simulink model "funcTest"  (R2020a)
settings: Solver=VariableStepAuto  StartTime=0.0  StopTime=10.0  RelTol=1e-3
settings Model: Creator=assem  LastModifiedBy=assem

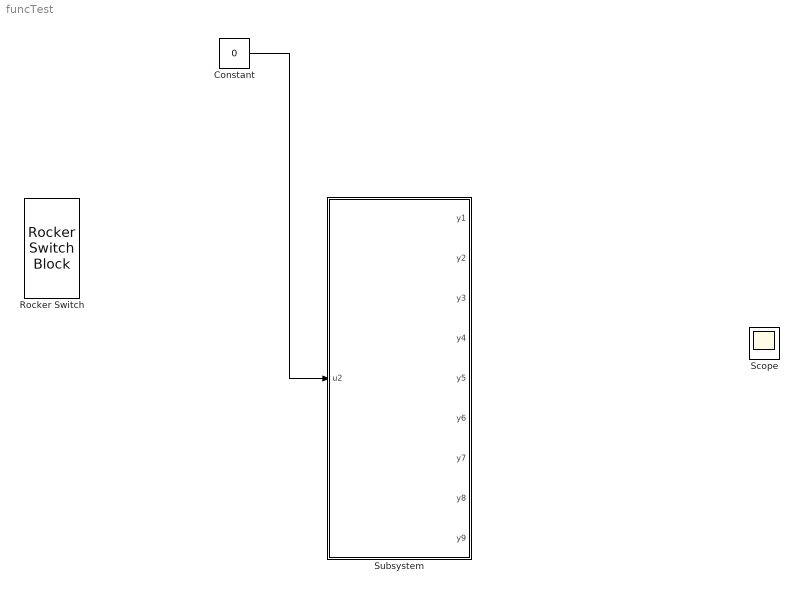
== system funcTest ==
  Constant : Constant  Value=0
  Rocker Switch : RockerSwitchBlock
      settings: Values={{'Off', 'On'}, [0 1]}
  Scope : Scope
  Subsystem : Subsystem
  wires:
  Constant/1 -> Subsystem/1(u2)

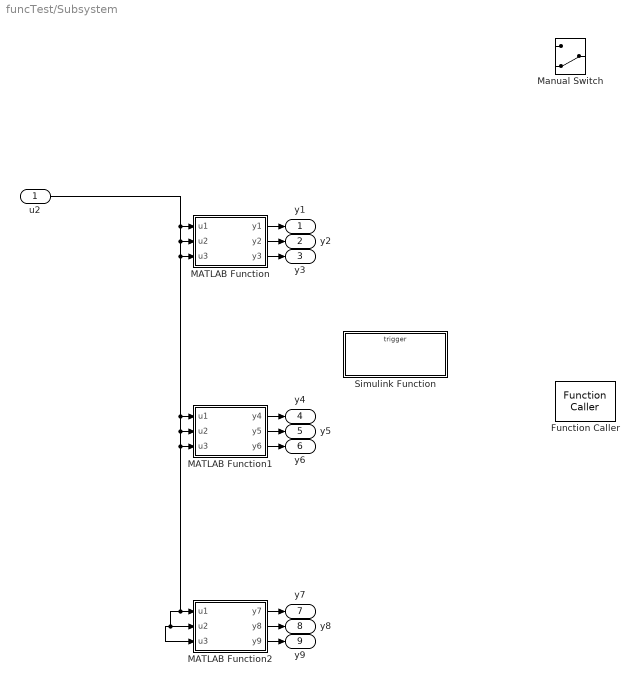
== system funcTest/Subsystem ==
  u2 : Inport
  Function Caller : FunctionCaller  FunctionPrototype=y = f(u)  InputArgumentSpecifications=<Enter example>  OutputArgumentSpecifications=<Enter example>
  MATLAB Function : MATLAB Function  TreatAsAtomicUnit=on
  MATLAB Function1 : MATLAB Function  TreatAsAtomicUnit=on
  MATLAB Function2 : MATLAB Function  TreatAsAtomicUnit=on
  Manual Switch : ManualSwitch  CurrentSetting=0
  Simulink Function : Subsystem  TreatAsAtomicUnit=on
  y1 : Outport
  y2 : Outport  Port=2
  y3 : Outport  Port=3
  y4 : Outport  Port=4
  y5 : Outport  Port=5
  y6 : Outport  Port=6
  y7 : Outport  Port=7
  y8 : Outport  Port=8
  y9 : Outport  Port=9
  wires:
  MATLAB Function2/2(y8) -> y8/1
  MATLAB Function1/1(y4) -> y4/1
  u2/1 -> MATLAB Function2/3(u3), MATLAB Function2/2(u2), MATLAB Function2/1(u1), MATLAB Function1/3(u3), MATLAB Function1/2(u2), MATLAB Function1/1(u1), MATLAB Function/3(u3), MATLAB Function/2(u2), MATLAB Function/1(u1)
  MATLAB Function2/1(y7) -> y7/1
  MATLAB Function2/3(y9) -> y9/1
  MATLAB Function/3(y3) -> y3/1
  MATLAB Function1/2(y5) -> y5/1
  MATLAB Function/1(y1) -> y1/1
  MATLAB Function1/3(y6) -> y6/1
  MATLAB Function/2(y2) -> y2/1

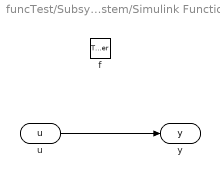
== system funcTest/Subsystem/Simulink Function ==
  f : TriggerPort  TriggerType=function-call  IsSimulinkFunction=on  FunctionName=f  FunctionVisibility=scoped  VariantControl=(inherit)
  u : ArgIn  DisableCoverage=on  ArgumentName=u
  y : ArgOut  DisableCoverage=on  ArgumentName=y
  wires:
  u/1 -> y/1

== matlab function funcTest/Subsystem/MATLAB Function1 ==
  data: u1 input; y4 output; u2 input; u3 input; y5 output; y6 output
function [y4, y5, y6] = fcn2(u1, u2, u3)
    
if (u1 == 1 && u3 == 1)
    y4 = 1;
    y5 = 0;
    y6 = 1;
else 
    y4 = 0;
    y5 = 0;
    y6 = 0;
end
end

== matlab function funcTest/Subsystem/MATLAB Function ==
  data: u1 input; y1 output; u2 input; u3 input; y2 output; y3 output
function [y1, y2, y3] = fcn1(u1, u2, u3)

if (u2 == 1 && u3 == 1)
    y1 = 0;
    y2 = 1;
    y3 = 1;
else 
    y1 = 0;
    y2 = 0;
    y3 = 0;
end
end

== matlab function funcTest/Subsystem/MATLAB Function2 ==
  data: u1 input; y7 output; u2 input; u3 input; y8 output; y9 output
function [y7, y8, y9] = fcn3(u1, u2, u3)

if (u1 == 1 && u2 == 1)
    y7 = 1;
    y8 = 1; 
    y9 = 0;

else 
    y7 = 0;
    y8 = 0;
    y9 = 0;
end
end
